simulink model "Quad_model"  (R2021b)
settings: Solver=VariableStepAuto  StartTime=0.0  StopTime=300  RelTol=1e-3
values from neighbouring files (symbols this model uses):
  A = c2d(A,1/500)    [FO_alpha.m]    (also in Model_Parameters.m = [gamma .* Wv .* (G_1+G_2) ; Wu]; wls.m = zeros(n_c,n_u))
  B = G_1+G_2    [Model_Parameters.m]    (also in wls_test.m)
  cd = 1    [Model_Parameters.m]
  G_1 = [ mot_eff,mot_eff,mot_eff,mot_eff;0,-12.8,0,12.8;2.7,0,-2.7,0;-0.115,0.115,-0.115,0.115]./conv    [Model_Parameters.m]    (also in wls_test.m)
  G_2 = [0,0,0,0;0,0,0,0;0,0,0,0;-0.06,0.06,-0.06,0.06]./conv    [Model_Parameters.m]    (also in wls_test.m)
  gamma = 10000    [Model_Parameters.m]    (also in full50.mat = [1 1 1 0]; wls_test.m = 100000000)
  gamma_o = 10000    [Model_Parameters.m]
  H_z_den = [1]    [Model_Parameters.m]
  H_z_num = [1]    [Model_Parameters.m]
  imax = 5    [Model_Parameters.m]    (also in wls_test.m)
  imax_o = 5    [Model_Parameters.m]
  M = 1    [Model_Parameters.m]
  mass = 2.339132*1    (= 2.339132)    [Model_Parameters.m]    (also in full50.mat = 3.5; pusher_effect.m)
  mot_den = [1]    [Model_Parameters.m]
  mot_num = [1]    [Model_Parameters.m]
  pseudo_g12 = pinv(G_1+G_2)    [Model_Parameters.m]    (also in wls_test.m)
  rho = 1.225    [Model_Parameters.m]    (also in full50.mat)
  Ts = 1/500    (= 0.002)    [Model_Parameters.m]
  uamax = 733    [Model_Parameters.m]    (also in wls_test.m)
  uamax_o = [0.4363,0.4363, 0]    [Model_Parameters.m]
  uamin_o = [-0.4363,-0.4363, mot_eff*4*733]    [Model_Parameters.m]
  up = [0,0,0,0]    [Model_Parameters.m]    (also in wls.m = umin; wls_test.m = [72,52,52,52])
  up_o = [0,0,0]    [Model_Parameters.m]
  v_lim = 10    [Model_Parameters.m]
  W_init = [0,0,0,0]    [Model_Parameters.m]    (also in wls_test.m)
  W_init_o = [0,0,0]    [Model_Parameters.m]
  weight = -g*mass    (= -22.94688492)    [Model_Parameters.m]
  Wu = [1, 0, 0, 0; 0, 1, 0, 0; 0, 0, 1, 0; 0, 0, 0, 1]    [Model_Parameters.m]    (also in wls_test.m = [1,1,1,1])
  Wu_o = [1,1,1]    [Model_Parameters.m]
  Wv = [100, 0, 0, 0; 0, 1000, 0, 0; 0, 0, 1000, 0; 0, 0, 0, 1 ]    [Model_Parameters.m]    (also in wls_test.m = [100,100,100,1])
  Wv_o = [1,1,1]    [Model_Parameters.m]
libraries: simulink x2, dspsrcs4 x1, sharedtransform x1, sim3dlib x1, uavsim3dlib x1, uavutilslib x1
settings Model: Creator=tomasodeponti  LastModifiedBy=Tomaso

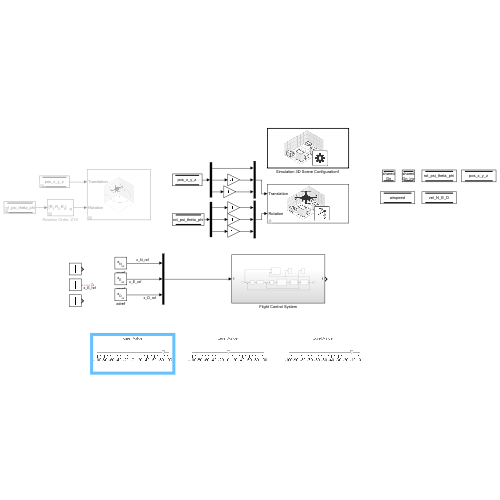
[thumbnail: Simulink's stored preview of the top-level diagram]
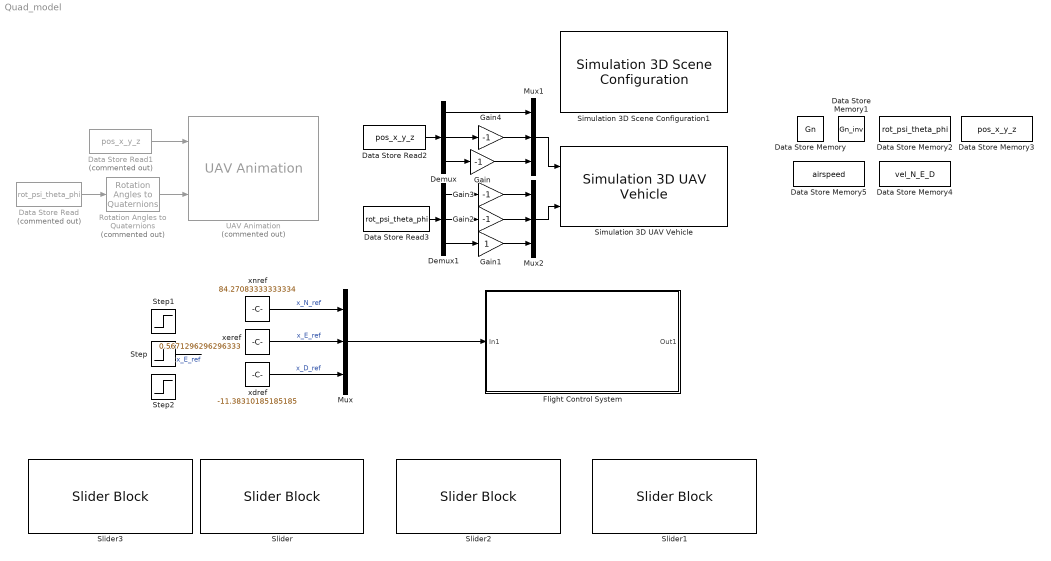
== system Quad_model ==
  Data Store Memory : DataStoreMemory  DataStoreName=Gn  ReadBeforeWriteMsg=warning  WriteAfterWriteMsg=warning  WriteAfterReadMsg=warning  InitialValue=[0,-9.81*mass,0;9.81*mass,0,0;0,0,1]  ShareAcrossModelInstances=on  ShowAdditionalParam=off  OutDataTypeStr=double  Dimensions=[3,3]
  Data Store Memory1 : DataStoreMemory  DataStoreName=Gn_inv  ReadBeforeWriteMsg=warning  WriteAfterWriteMsg=warning  WriteAfterReadMsg=warning  InitialValue=[0,-1/weight,0;1/weight,0,0;0,0,1]  ShareAcrossModelInstances=on  ShowAdditionalParam=off  OutDataTypeStr=double  Dimensions=[3,3]
  Data Store Memory2 : DataStoreMemory  DataStoreName=rot_psi_theta_phi  ReadBeforeWriteMsg=warning  WriteAfterWriteMsg=warning  WriteAfterReadMsg=warning  InitialValue=[0,0,0]  ShowAdditionalParam=off  OutDataTypeStr=double
  Data Store Memory3 : DataStoreMemory  DataStoreName=pos_x_y_z  ReadBeforeWriteMsg=warning  WriteAfterWriteMsg=warning  WriteAfterReadMsg=warning  InitialValue=[0,0,0]  ShowAdditionalParam=off  OutDataTypeStr=double
  Data Store Memory4 : DataStoreMemory  DataStoreName=vel_N_E_D  ReadBeforeWriteMsg=warning  WriteAfterWriteMsg=warning  WriteAfterReadMsg=warning  InitialValue=[0,0,0]  ShowAdditionalParam=off  OutDataTypeStr=double
  Data Store Memory5 : DataStoreMemory  DataStoreName=airspeed  ReadBeforeWriteMsg=warning  WriteAfterWriteMsg=warning  WriteAfterReadMsg=warning  InitialValue=[0]  ShowAdditionalParam=off  OutMin=[0]  OutDataTypeStr=double
  Data Store Read : DataStoreRead  Commented=on  DataStoreName=rot_psi_theta_phi  IndexOptions=Index vector (dialog)  Indices=1  OutputSizes=1
  Data Store Read1 : DataStoreRead  Commented=on  DataStoreName=pos_x_y_z  IndexOptions=Index vector (dialog)  Indices=1  OutputSizes=1
  Data Store Read2 : DataStoreRead  DataStoreName=pos_x_y_z  IndexOptions=Index vector (dialog)  Indices=1  OutputSizes=1
  Data Store Read3 : DataStoreRead  DataStoreName=rot_psi_theta_phi  IndexOptions=Index vector (dialog)  Indices=1  OutputSizes=1
  Demux : Demux  Outputs=3
  Demux1 : Demux  Outputs=3
  Flight Control System : Subsystem
  Gain{,2..4} (4 alike) : Gain  Gain=-1
  Gain1 : Gain
  Mux : Mux  Inputs=3
  Mux1 : Mux  Inputs=3
  Mux2 : Mux  Inputs=3
  Rotation Angles to Quaternions : sharedtransform/Rotation Angles to Quaternions  Commented=on  rotationOrder=ZYX  aMode=aMode
      settings: SourceProductBaseCode=AE,PW,DR,MT,UV,VE
  Simulation 3D Scene Configuration1 : sim3dlib/Simulation 3D Scene Configuration  Priority=0  ProjectFormat_internal=Default Scenes  ProjectFormat=Default Scenes  SceneDesc=US city block  ProjectName=C:\Program Files\MATLAB\R2021b\toolbox\shared\sim3d_projects\automotive_project\UE4\WindowsNoEditor\VehicleSimulation.exe  ScenePath=/Game/Maps/USCityBlock  vehTagList={'Scene Origin';'SimulinkVehicle1'}  vehTag=SimulinkVehicle1  OpVisEn=off  Ts=1/60  EnableWindow=on  EnableWeather=off  SunAltitude=40.0  SunAzimuth=90  clouds=10  wind=1  fog=0  rain=0  sensorTag=MainCamera2  sensorId=2  sensorName=MainCamera2  mountLoc=Origin  offsetFlag=off  tmountOffset=[0, 0, 0]  rmountOffset=[0, 0, 0]  HorizontalResolution=1280  VerticalResolution=720  HorizontalFOV=60  mountPoint=[0 0 0]  mountOrientation=[0 0 0]  aMode=4  ID=2
      settings: SourceProductBaseCode=AE,DR,UV,VE
  Simulation 3D UAV Vehicle : uavsim3dlib/Simulation 3D UAV Vehicle  Priority=-1  Mesh=Quadrotor  MeshPath=/MathWorksUAVContent/UAVs/HexaRotorUAV/HexaRotor.HexaRotor  Color=Black  ActorName=SimulinkVehicle1  InitialTranslation=[0 0 5]  InitialRotation=[0 0 0]  SampleTime=-1  ActorType=SimulinkVehicle  ID=1  aMode=4  ActorTag=SimulinkVehicle1
      settings: SourceProductBaseCode=UV
  Slider : SliderBlock  ScaleMin=-100
  Slider1 : SliderBlock  ScaleMin=-100  ScaleMax=0
  Slider2 : SliderBlock  ScaleMin=-100
  Slider3 : SliderBlock  ScaleMin=-3.14  ScaleMax=3.14
  Step : Step  Time=3  After=50  SampleTime=0
  Step1 : Step  Time=3  After=100  SampleTime=0
  Step2 : Step  Time=4  After=-25  SampleTime=0
  UAV Animation : uavutilslib/UAV Animation  Commented=on  UAVType=Multirotor  UAVSize=1  InertialZDirection=Down  SampleTime=-1
      settings: SourceProductBaseCode=UV
  xdref : Constant  Value=-11.38310185185185  SampleTime=Ts
      mask Display: disp('x_{D_{ref}}','texmode','on')
  xeref : Constant  Value=0.5671296296296333  SampleTime=Ts
      mask Display: disp('x_{E_{ref}}','texmode','on')
  xnref : Constant  Value=84.27083333333334  SampleTime=Ts
      mask Display: disp('x_{N_{ref}}','texmode','on')
  wires:
  Data Store Read1/1 -> UAV Animation/1
  Data Store Read/1 -> Rotation Angles to Quaternions/1
  Rotation Angles to Quaternions/1 -> UAV Animation/2
  xdref/1 -> Mux/3  "x_D_ref"
  xnref/1 -> Mux/1  "x_N_ref"
  Mux/1 -> Flight Control System/1(In1)
  xeref/1 -> Mux/2  "x_E_ref"
  Step/1 -> ?  "x_E_ref"
  Data Store Read2/1 -> Demux/1
  Mux1/1 -> Simulation 3D UAV Vehicle/1
  Demux/3 -> Gain/1
  Gain/1 -> Mux1/3
  Data Store Read3/1 -> Demux1/1
  Demux1/3 -> Gain1/1
  Gain1/1 -> Mux2/3
  Mux2/1 -> Simulation 3D UAV Vehicle/2
  Demux1/2 -> Gain2/1
  Gain2/1 -> Mux2/2
  Demux1/1 -> Gain3/1
  Gain3/1 -> Mux2/1
  Demux/2 -> Gain4/1
  Gain4/1 -> Mux1/2
  Demux/1 -> Mux1/1

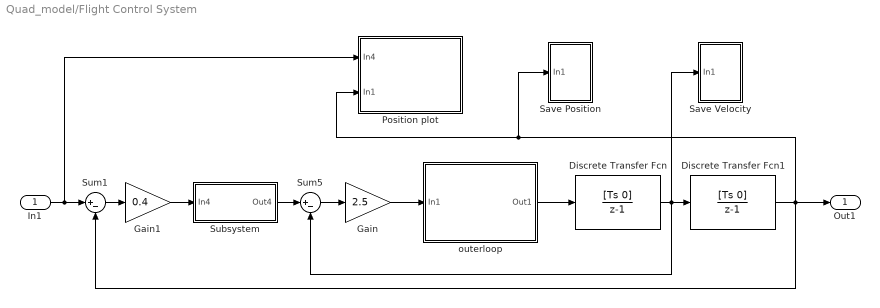
== system Quad_model/Flight Control System ==
  In1 : Inport
  Discrete Transfer Fcn : DiscreteTransferFcn  Numerator=[Ts 0]  Denominator=[1 -1]
  Discrete Transfer Fcn1 : DiscreteTransferFcn  Numerator=[Ts 0]  Denominator=[1 -1]
  Gain : Gain  Gain=2.5
      mask Display: disp('K_{u}','texmode','on')
  Gain1 : Gain  Gain=0.4
      mask Display: disp('K_\xi','texmode','on')
  Position plot : Subsystem
  Save Position : Subsystem
  Save Velocity : Subsystem
  Subsystem : Subsystem
      mask Display: disp('Velocity lim')
  Sum1 : Sum  Inputs=|+-
  Sum5 : Sum  Inputs=|+-
  outerloop : Subsystem
  Out1 : Outport
  wires:
  outerloop/1(Out1) -> Discrete Transfer Fcn/1
  Discrete Transfer Fcn1/1 -> Position plot/2(In1), Save Position/1(In1), Out1/1, Sum1/2
  Sum5/1 -> Gain/1
  Gain/1 -> outerloop/1(In1)
  Discrete Transfer Fcn/1 -> Save Velocity/1(In1), Sum5/2, Discrete Transfer Fcn1/1
  In1/1 -> Position plot/1(In4), Sum1/1
  Gain1/1 -> Subsystem/1(In4)
  Subsystem/1(Out4) -> Sum5/1
  Sum1/1 -> Gain1/1

== system Quad_model/Flight Control System/Position plot ==
  In4 : Inport
  In1 : Inport  Port=2
  Demux : Demux  Outputs=3
  Demux1 : Demux  Outputs=3
  Mux : Mux  Inputs=2
  Mux1 : Mux  Inputs=2
  Mux3 : Mux  Inputs=2
  Position Plotter : Scope  NumInputPorts=3
  wires:
  Demux/3 -> Mux3/1  "x_D"
  Demux/2 -> Mux1/1  "x_E"
  In1/1 -> Demux/1
  Mux/1 -> Position Plotter/1
  Demux/1 -> Mux/1  "x_N"
  Mux1/1 -> Position Plotter/2
  Mux3/1 -> Position Plotter/3
  In4/1 -> Demux1/1
  Demux1/1 -> Mux/2  "x_N_ref"
  Demux1/2 -> Mux1/2  "x_E_ref"
  Demux1/3 -> Mux3/2  "x_D_ref"

== system Quad_model/Flight Control System/Save Position ==
  In1 : Inport
  Data Store Write : DataStoreWrite  DataStoreName=pos_x_y_z  IndexOptions=Index vector (dialog)  Indices=1  OutputSizes=1
  Demux : Demux  Outputs=3
  Mux4 : Mux  Inputs=3
  wires:
  Mux4/1 -> Data Store Write/1
  Demux/2 -> Mux4/2
  Demux/1 -> Mux4/1
  Demux/3 -> Mux4/3
  In1/1 -> Demux/1

== system Quad_model/Flight Control System/Save Velocity ==
  In1 : Inport
  Data Store Write : DataStoreWrite  DataStoreName=vel_N_E_D  IndexOptions=Index vector (dialog)  Indices=1  OutputSizes=1
  Data Store Write1 : DataStoreWrite  DataStoreName=airspeed  IndexOptions=Index vector (dialog)  Indices=1  OutputSizes=1
  Demux : Demux  Outputs=3
  Dot Product : DotProduct  InputSameDT=on  OutDataTypeStr=Inherit: Inherit via internal rule
  Mux : Mux  Inputs=2
  Mux4 : Mux  Inputs=3
  Scope : Scope
  Square Root : Sqrt  SaturateOnIntegerOverflow=on
  wires:
  Mux4/1 -> Data Store Write/1
  Demux/2 -> Mux/2, Mux4/2
  Demux/1 -> Mux/1, Mux4/1
  Demux/3 -> Mux4/3
  In1/1 -> Demux/1
  Dot Product/1 -> Square Root/1
  Square Root/1 -> Scope/1, Data Store Write1/1
  Mux/1 -> Dot Product/2, Dot Product/1

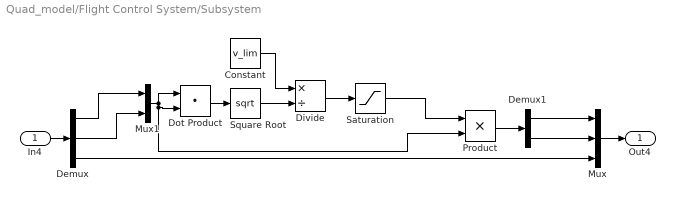
== system Quad_model/Flight Control System/Subsystem ==
  In4 : Inport
  Constant : Constant  Value=v_lim
  Demux : Demux  Outputs=3
  Demux1 : Demux  Outputs=2
  Divide : Product  Inputs=*/
  Dot Product : DotProduct  InputSameDT=on  OutDataTypeStr=Inherit: Inherit via internal rule
  Mux : Mux  Inputs=3
  Mux1 : Mux  Inputs=2
  Product : Product
  Saturation : Saturate  UpperLimit=1  LowerLimit=0
  Square Root : Sqrt  SaturateOnIntegerOverflow=on
  Out4 : Outport
  wires:
  In4/1 -> Demux/1
  Mux/1 -> Out4/1
  Constant/1 -> Divide/1
  Demux/3 -> Mux/3
  Demux/1 -> Mux1/1
  Demux/2 -> Mux1/2
  Dot Product/1 -> Square Root/1
  Mux1/1 -> Product/2, Dot Product/2, Dot Product/1
  Square Root/1 -> Divide/2
  Divide/1 -> Saturation/1
  Product/1 -> Demux1/1
  Demux1/1 -> Mux/1
  Demux1/2 -> Mux/2
  Saturation/1 -> Product/1

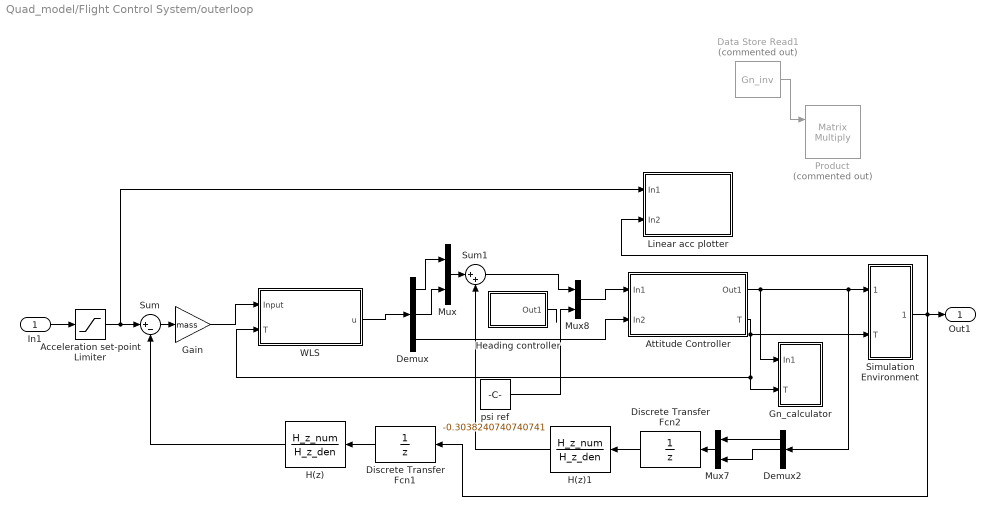
== system Quad_model/Flight Control System/outerloop ==
  In1 : Inport
  Acceleration set-point Limiter : Saturate  UpperLimit=[3,3,3]  LowerLimit=[-3,-3,-3]
  Attitude Controller : Subsystem
  Data Store Read1 : DataStoreRead  Commented=on  DataStoreName=Gn_inv  SampleTime=Ts  IndexOptions=Index vector (dialog)  Indices=1  OutputSizes=1
  Demux : Demux  Outputs=3
  Demux2 : Demux  Outputs=3
  Discrete Transfer Fcn1 : DiscreteTransferFcn  Denominator=[1 0]
  Discrete Transfer Fcn2 : DiscreteTransferFcn  Denominator=[1 0]
  Gain : Gain  Gain=mass
  Gn_calculator : Subsystem
  H(z) : DiscreteTransferFcn  Numerator=H_z_num  Denominator=H_z_den  DenCoefDataTypeStr=int16
      mask Display: disp('H(z)')
  H(z)1 : DiscreteTransferFcn  Numerator=H_z_num  Denominator=H_z_den  DenCoefDataTypeStr=int16
      mask Display: disp('H(z)')
  Heading controller : Subsystem
  Linear acc plotter : Subsystem
  Mux : Mux  Inputs=2
  Mux7 : Mux  Inputs=2
  Mux8 : Mux  Inputs=2
  Product : Product  Commented=on  Multiplication=Matrix(*)
      mask Display: disp('G(\eta_0,T_0)^+','texmode','on')
  Simulation Environment : Subsystem
  Sum : Sum  Inputs=|+-
  Sum1 : Sum  Inputs=|++
  WLS : Subsystem
  psi ref : Constant  Value=-0.3038240740740741
  Out1 : Outport
  wires:
  Mux7/1 -> Discrete Transfer Fcn2/1
  Data Store Read1/1 -> Product/1
  WLS/1(u) -> Demux/1
  Discrete Transfer Fcn2/1 -> H(z)1/1
  Mux/1 -> Sum1/1
  Demux/3 -> Attitude Controller/2(In2)
  Attitude Controller/1(Out1) -> Gn_calculator/1(In1), Demux2/1, Simulation Environment/1(In1)
  H(z)/1 -> Sum/2
  Discrete Transfer Fcn1/1 -> H(z)/1
  Gain/1 -> WLS/1(Input)
  Demux/2 -> Mux/2
  Sum/1 -> Gain/1
  Attitude Controller/2(T) -> WLS/2(T), Gn_calculator/2(T), Simulation Environment/2(T)
  Sum1/1 -> Mux8/1
  Mux8/1 -> Attitude Controller/1(In1)
  Demux2/1 -> Mux7/1
  H(z)1/1 -> Sum1/2
  Demux/1 -> Mux/1
  Simulation Environment/1(Out1) -> Discrete Transfer Fcn1/1, Out1/1, Linear acc plotter/2(In2)
  Demux2/2 -> Mux7/2
  Acceleration set-point Limiter/1 -> Linear acc plotter/1(In1), Sum/1
  In1/1 -> Acceleration set-point Limiter/1
  psi ref/1 -> Mux8/2
  Heading controller/1(Out1) -> ?

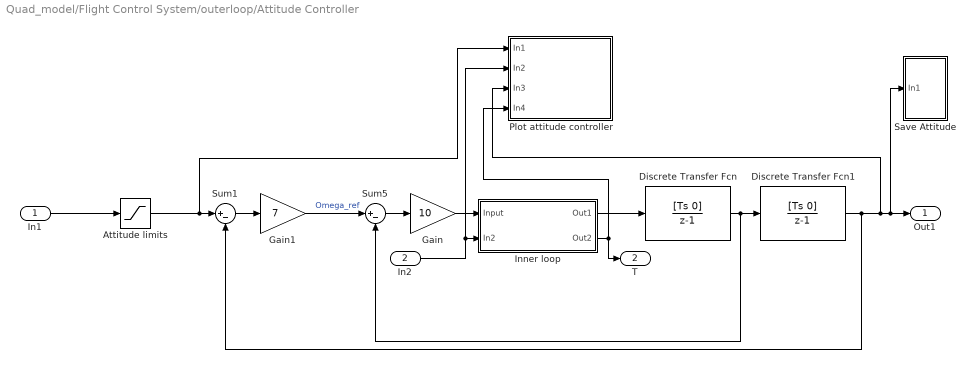
== system Quad_model/Flight Control System/outerloop/Attitude Controller ==
  In1 : Inport
  In2 : Inport  Port=2
  Attitude limits : Saturate  UpperLimit=[25,25,180]*pi/180  LowerLimit=[-25,-25,-180]*pi/180
  Discrete Transfer Fcn : DiscreteTransferFcn  Numerator=[Ts 0]  Denominator=[1 -1]
  Discrete Transfer Fcn1 : DiscreteTransferFcn  Numerator=[Ts 0]  Denominator=[1 -1]
  Gain : Gain  Gain=10
      mask Display: disp('K_\Omega','texmode','on')
  Gain1 : Gain  Gain=7
      mask Display: disp('K_\eta','texmode','on')
  Inner loop : Subsystem
  Plot attitude controller : Subsystem
  Save Attitude : Subsystem
  Sum1 : Sum  Inputs=|+-
  Sum5 : Sum  Inputs=|+-
  Out1 : Outport
  T : Outport  Port=2
  wires:
  Gain1/1 -> Sum5/1  "Omega_ref"
  Sum5/1 -> Gain/1
  Sum1/1 -> Gain1/1
  Discrete Transfer Fcn/1 -> Sum5/2, Discrete Transfer Fcn1/1
  Gain/1 -> Inner loop/1(Input)
  Inner loop/1(Out1) -> Discrete Transfer Fcn/1
  Discrete Transfer Fcn1/1 -> Plot attitude controller/3(In3), Save Attitude/1(In1), Out1/1, Sum1/2
  Inner loop/2(Out2) -> T/1, Plot attitude controller/4(In4)
  In2/1 -> Plot attitude controller/2(In2), Inner loop/2(In2)
  Attitude limits/1 -> Plot attitude controller/1(In1), Sum1/1
  In1/1 -> Attitude limits/1

== system Quad_model/Flight Control System/outerloop/Gn_calculator ==
  In1 : Inport
  T : Inport  Port=2
  Constant : Constant  Value=weight
  Demux : Demux  Outputs=3
  Gn : MATLAB Function  TreatAsAtomicUnit=on
  Gn_inv : MATLAB Function  TreatAsAtomicUnit=on
  wires:
  Demux/1 -> Gn_inv/2(phi), Gn/2(phi)
  In1/1 -> Demux/1
  T/1 -> Gn_inv/1(T), Gn/1(T)
  Demux/2 -> Gn_inv/3(theta), Gn/3(theta)
  Demux/3 -> Gn_inv/4(psi), Gn/4(psi)

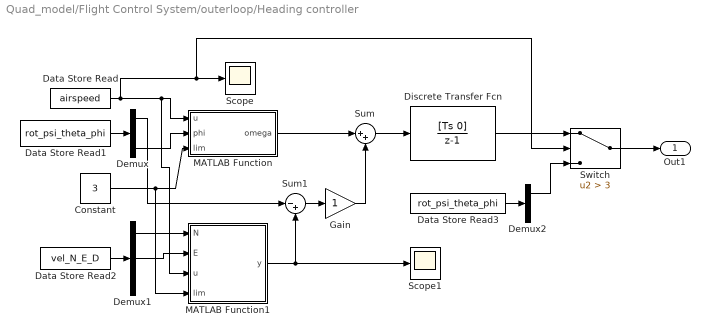
== system Quad_model/Flight Control System/outerloop/Heading controller ==
  Constant : Constant  Value=3
  Data Store Read : DataStoreRead  DataStoreName=airspeed  IndexOptions=Index vector (dialog)  Indices=1  OutputSizes=1
  Data Store Read1 : DataStoreRead  DataStoreName=rot_psi_theta_phi  IndexOptions=Index vector (dialog)  Indices=1  OutputSizes=1
  Data Store Read2 : DataStoreRead  DataStoreName=vel_N_E_D  IndexOptions=Index vector (dialog)  Indices=1  OutputSizes=1
  Data Store Read3 : DataStoreRead  DataStoreName=rot_psi_theta_phi  IndexOptions=Index vector (dialog)  Indices=1  OutputSizes=1
  Demux : Demux  Outputs=3
  Demux1 : Demux  Outputs=3
  Demux2 : Demux  Outputs=3
  Discrete Transfer Fcn : DiscreteTransferFcn  Numerator=[Ts 0]  Denominator=[1 -1]
  Gain : Gain
  MATLAB Function : MATLAB Function  TreatAsAtomicUnit=on
  MATLAB Function1 : MATLAB Function  TreatAsAtomicUnit=on
  Scope : Scope
  Scope1 : Scope
  Sum : Sum  Inputs=|++
  Sum1 : Sum  Inputs=|-+
  Switch : Switch  Criteria=u2 > Threshold  Threshold=3
  Out1 : Outport
  wires:
  Data Store Read1/1 -> Demux/1
  Demux/3 -> MATLAB Function/2(phi)
  Data Store Read/1 -> Switch/2, Scope/1, MATLAB Function1/3(u), MATLAB Function/1(u)
  Data Store Read2/1 -> Demux1/1
  Demux1/1 -> MATLAB Function1/1(N)
  Demux1/2 -> MATLAB Function1/2(E)
  Switch/1 -> Out1/1
  Sum/1 -> Discrete Transfer Fcn/1
  MATLAB Function/1(omega) -> Sum/1
  Gain/1 -> Sum/2
  MATLAB Function1/1(y) -> Sum1/2, Scope1/1
  Demux/1 -> Sum1/1
  Sum1/1 -> Gain/1
  Constant/1 -> MATLAB Function/3(lim), MATLAB Function1/4(lim)
  Discrete Transfer Fcn/1 -> Switch/1
  Data Store Read3/1 -> Demux2/1
  Demux2/1 -> Switch/3

== system Quad_model/Flight Control System/outerloop/Linear acc plotter ==
  In1 : Inport
  In2 : Inport  Port=2
  Constant1 : Constant  Value=0  SampleTime=Ts
      mask Display: disp('a_{N_{ref}}','texmode','on')
  Constant2 : Constant  Value=0  SampleTime=Ts
      mask Display: disp('a_{E_{ref}}','texmode','on')
  Constant3 : Constant  Value=0  SampleTime=Ts
      mask Display: disp('a_{D_{ref}}','texmode','on')
  Demux1 : Demux  Outputs=3
  Demux2 : Demux  Outputs=3
  Mux1 : Mux  Inputs=2
  Mux2 : Mux  Inputs=3
  Mux3 : Mux  Inputs=2
  Mux4 : Mux  Inputs=2
  Scope : Scope  NumInputPorts=3
  wires:
  Demux1/3 -> Mux4/1  "a_D"
  Mux1/1 -> Scope/1
  In2/1 -> Demux1/1
  Mux3/1 -> Scope/2
  Mux4/1 -> Scope/3
  Demux1/2 -> Mux3/1  "a_E"
  Demux1/1 -> Mux1/1  "a_N"
  Constant2/1 -> Mux2/2  "a_E_ref"
  Constant1/1 -> Mux2/1  "a_N_ref"
  Constant3/1 -> Mux2/3  "a_D_ref"
  In1/1 -> Demux2/1
  Demux2/1 -> Mux1/2  "a_N_ref"
  Demux2/2 -> Mux3/2  "a_E_ref"
  Demux2/3 -> Mux4/2  "a_D_ref"

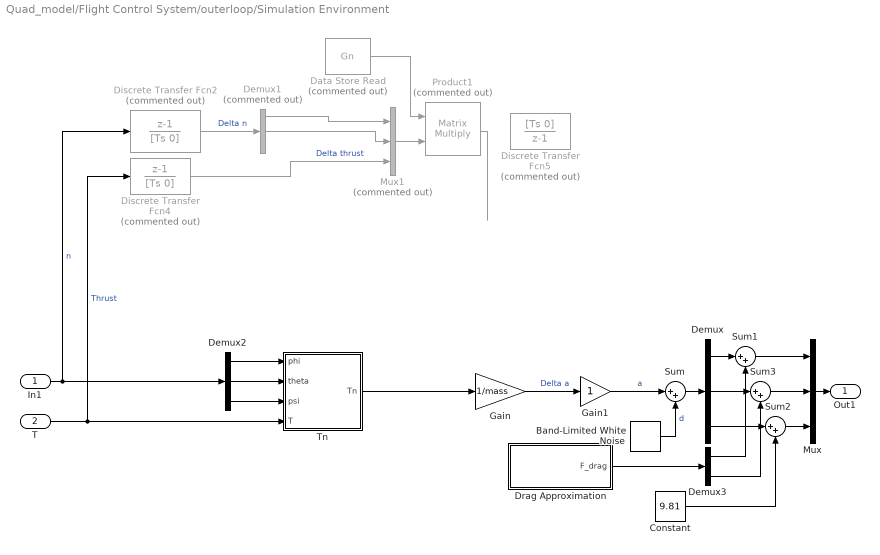
== system Quad_model/Flight Control System/outerloop/Simulation Environment ==
  In1 : Inport
  T : Inport  Port=2
  Band-Limited White Noise : simulink/Sources/Band-Limited White Noise  Cov=[0.00000001]  Ts=Ts  seed=[23341]
  Constant : Constant  Value=9.81
  Data Store Read : DataStoreRead  Commented=on  DataStoreName=Gn  IndexOptions=Index vector (dialog)  Indices=1  OutputSizes=1
  Demux : Demux  Outputs=3
  Demux1 : Demux  Commented=on  Outputs=3
  Demux2 : Demux  Outputs=3
  Demux3 : Demux  Outputs=2
  Discrete Transfer Fcn2 : DiscreteTransferFcn  Commented=on  Numerator=[1 -1]  Denominator=[Ts 0]
  Discrete Transfer Fcn4 : DiscreteTransferFcn  Commented=on  Numerator=[1 -1]  Denominator=[Ts 0]
  Discrete Transfer Fcn5 : DiscreteTransferFcn  Commented=on  Numerator=[Ts 0]  Denominator=[1 -1]
  Drag Approximation : Subsystem
  Gain : Gain  Gain=1/mass
  Gain1 : Gain
  Mux : Mux  Inputs=3
  Mux1 : Mux  Commented=on  Inputs=3
  Product1 : Product  Commented=on  Multiplication=Matrix(*)
      mask Display: disp('G(\eta_0,T_0)','texmode','on')
  Sum{,1..3} (4 alike) : Sum  Inputs=|++
  Tn : MATLAB Function  TreatAsAtomicUnit=on
  Out1 : Outport
  wires:
  In1/1 -> Discrete Transfer Fcn2/1, Demux2/1  "n"
  Data Store Read/1 -> Product1/1
  Mux1/1 -> Product1/2
  Demux1/1 -> Mux1/1
  Demux1/2 -> Mux1/2
  Discrete Transfer Fcn2/1 -> Demux1/1  "Delta n"
  Gain/1 -> Gain1/1  "Delta a"
  Gain1/1 -> Sum/1  "a"
  Product1/1 -> ?
  T/1 -> Discrete Transfer Fcn4/1, Tn/4(T)  "Thrust"
  Discrete Transfer Fcn4/1 -> Mux1/3  "Delta thrust"
  Band-Limited White Noise/1 -> Sum/2  "d"
  Demux2/1 -> Tn/1(phi)
  Demux2/2 -> Tn/2(theta)
  Demux2/3 -> Tn/3(psi)
  Tn/1(Tn) -> Gain/1
  Drag Approximation/1(F_drag) -> Demux3/1
  Sum/1 -> Demux/1
  Sum3/1 -> Mux/2
  Mux/1 -> Out1/1
  Demux/3 -> Sum2/1
  Sum2/1 -> Mux/3
  Sum1/1 -> Mux/1
  Demux/1 -> Sum1/1
  Demux/2 -> Sum3/1
  Demux3/1 -> Sum1/2
  Demux3/2 -> Sum3/2
  Constant/1 -> Sum2/2

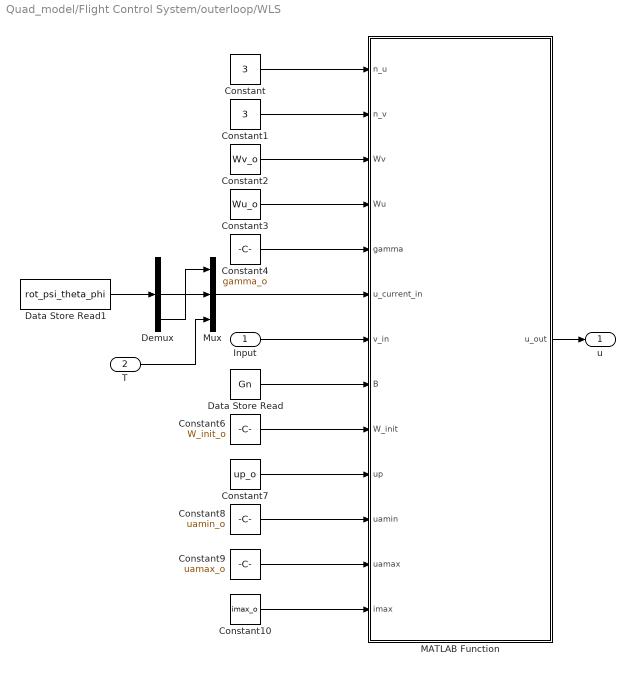
== system Quad_model/Flight Control System/outerloop/WLS ==
  Input : Inport
  T : Inport  Port=2
  Constant : Constant  Value=3
  Constant1 : Constant  Value=3
  Constant10 : Constant  Value=imax_o
  Constant2 : Constant  Value=Wv_o
  Constant3 : Constant  Value=Wu_o
  Constant4 : Constant  Value=gamma_o
  Constant6 : Constant  Value=W_init_o
  Constant7 : Constant  Value=up_o
  Constant8 : Constant  Value=uamin_o
  Constant9 : Constant  Value=uamax_o
  Data Store Read : DataStoreRead  DataStoreName=Gn  IndexOptions=Index vector (dialog)  Indices=1  OutputSizes=1
  Data Store Read1 : DataStoreRead  DataStoreName=rot_psi_theta_phi  IndexOptions=Index vector (dialog)  Indices=1  OutputSizes=1
  Demux : Demux  Outputs=3
  MATLAB Function : MATLAB Function  TreatAsAtomicUnit=on
  Mux : Mux  Inputs=3
  u : Outport
  wires:
  Constant8/1 -> MATLAB Function/11(uamin)
  Constant4/1 -> MATLAB Function/5(gamma)
  Constant/1 -> MATLAB Function/1(n_u)
  MATLAB Function/1(u_out) -> u/1
  Data Store Read/1 -> MATLAB Function/8(B)
  Constant9/1 -> MATLAB Function/12(uamax)
  Constant6/1 -> MATLAB Function/9(W_init)
  Constant10/1 -> MATLAB Function/13(imax)
  Constant1/1 -> MATLAB Function/2(n_v)
  Constant2/1 -> MATLAB Function/3(Wv)
  Constant3/1 -> MATLAB Function/4(Wu)
  Constant7/1 -> MATLAB Function/10(up)
  Mux/1 -> MATLAB Function/6(u_current_in)
  Input/1 -> MATLAB Function/7(v_in)
  Data Store Read1/1 -> Demux/1
  Demux/3 -> Mux/1
  Demux/2 -> Mux/2
  T/1 -> Mux/3

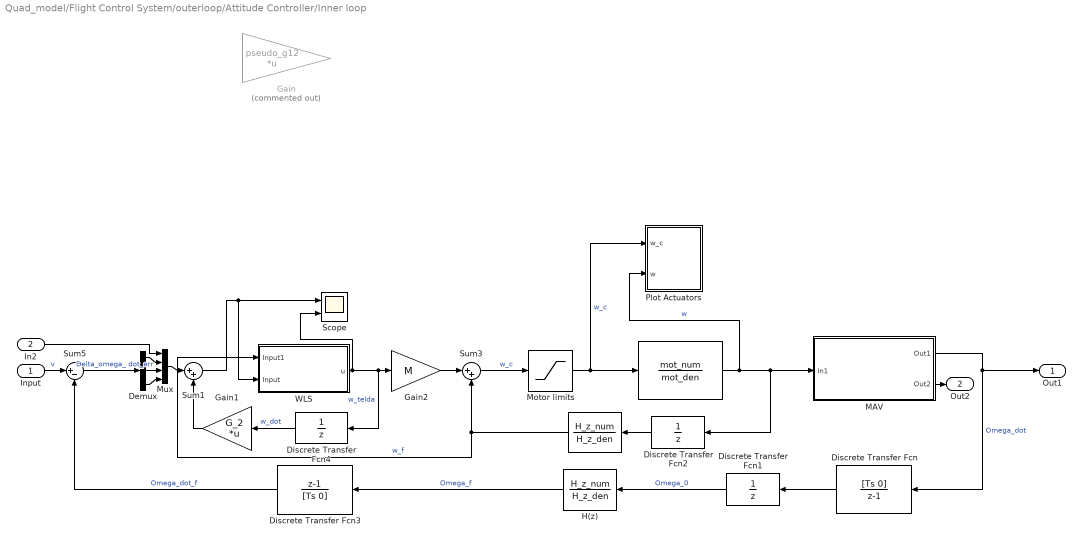
== system Quad_model/Flight Control System/outerloop/Attitude Controller/Inner loop ==
  Input : Inport  PortDimensions=3
  In2 : Inport  Port=2
  " " : DiscreteTransferFcn  Numerator=H_z_num  Denominator=H_z_den  DenCoefDataTypeStr=int16
      mask Display: disp('H(z)')
  "  " : DiscreteTransferFcn  Numerator=mot_num  Denominator=mot_den  DenCoefDataTypeStr=int16
      mask Display: disp('A(z)')
  Demux : Demux  Outputs=3
  Discrete Transfer Fcn : DiscreteTransferFcn  Numerator=[Ts 0]  Denominator=[1 -1]
  Discrete Transfer Fcn1 : DiscreteTransferFcn  Denominator=[1 0]
  Discrete Transfer Fcn2 : DiscreteTransferFcn  Denominator=[1 0]
  Discrete Transfer Fcn3 : DiscreteTransferFcn  Numerator=[1 -1]  Denominator=[Ts 0]
  Discrete Transfer Fcn4 : DiscreteTransferFcn  Denominator=[1 0]
  Gain : Gain  Commented=on  Gain=pseudo_g12  Multiplication=Matrix(K*u)
      mask Display: disp('(G1+G2)^+','texmode','on')
  Gain1 : Gain  Gain=G_2  Multiplication=Matrix(K*u)
      mask Display: disp('G2')
  Gain2 : Gain  Gain=M
      mask Display: disp('M')
  H(z) : DiscreteTransferFcn  Numerator=H_z_num  Denominator=H_z_den  DenCoefDataTypeStr=int16
      mask Display: disp('H(z)')
  MAV : Subsystem
      mask Display:
      | %image('C:\Users\Tomaso\Pictures\Screenshots\Screenshot 2021-12-02 165056.png'); % Use "Edit Image" on toolstrip to change.
      | disp('MAV')
  Motor limits : Saturate  UpperLimit=733  LowerLimit=52
  Mux : Mux
  Plot Actuators : Subsystem
  Scope : Scope  NumInputPorts=2
  Sum1 : Sum  Inputs=|++
  Sum3 : Sum  Inputs=|++
  Sum5 : Sum  Inputs=|+-
  WLS : Subsystem
  Out1 : Outport  PortDimensions=3
  Out2 : Outport  Port=2
  wires:
  "  "/1 -> Plot Actuators/2(w), Discrete Transfer Fcn2/1, MAV/1(In1)  "w"
  Discrete Transfer Fcn/1 -> Discrete Transfer Fcn1/1
  Discrete Transfer Fcn1/1 -> H(z)/1  "Omega_0"
  Discrete Transfer Fcn2/1 -> " "/1
  Motor limits/1 -> Plot Actuators/1(w_c), "  "/1  "w_c"
  " "/1 -> Sum3/2, WLS/1(Input1)  "w_f"
  H(z)/1 -> Discrete Transfer Fcn3/1  "Omega_f"
  Discrete Transfer Fcn3/1 -> Sum5/2  "Omega_dot_f"
  WLS/1(u) -> Scope/2, Discrete Transfer Fcn4/1, Gain2/1  "w_telda"
  Sum5/1 -> Demux/1  "Delta_omega_ dot_err"
  Sum1/1 -> Scope/1, WLS/2(Input)
  Discrete Transfer Fcn4/1 -> Gain1/1  "w_dot"
  Gain1/1 -> Sum1/2
  Input/1 -> Sum5/1  "v"
  Gain2/1 -> Sum3/1
  Sum3/1 -> Motor limits/1  "w_c"
  MAV/1(Out1) -> Discrete Transfer Fcn/1, Out1/1  "Omega_dot"
  In2/1 -> Mux/1
  Mux/1 -> Sum1/1
  Demux/1 -> Mux/2
  Demux/2 -> Mux/3
  Demux/3 -> Mux/4
  MAV/2(Out2) -> Out2/1

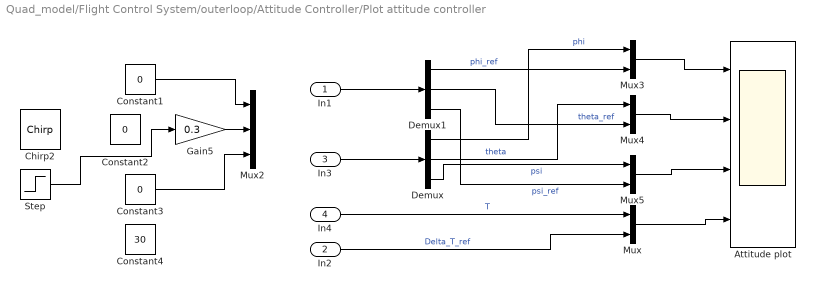
== system Quad_model/Flight Control System/outerloop/Attitude Controller/Plot attitude controller ==
  In1 : Inport
  In2 : Inport  Port=2
  In3 : Inport  Port=3
  In4 : Inport  Port=4
  Attitude plot : Scope  NumInputPorts=4
  Chirp2 : dspsrcs4/Chirp  sweep=Linear  mode=Unidirectional  f0=0.1  f1=0.5  t1=1  Tsweep=10  phase=0  Ts=Ts  spf=1  datatype=Double  OutputFrames=off
  Constant1 : Constant  Value=0
      mask Display: disp('\phi_{ref}','texmode','on')
  Constant2 : Constant  Value=0
      mask Display: disp('\theta_{ref}','texmode','on')
  Constant3 : Constant  Value=0
      mask Display: disp('\psi_{ref}','texmode','on')
  Constant4 : Constant  Value=30
      mask Display: disp('\Delta T','texmode','on')
  Demux : Demux  Outputs=3
  Demux1 : Demux  Outputs=3
  Gain5 : Gain  Gain=0.3
  Mux{,3..5} (4 alike) : Mux  Inputs=2
  Mux2 : Mux  Inputs=3
  Step : Step  SampleTime=0
  wires:
  In4/1 -> Mux/1  "T"
  In3/1 -> Demux/1
  Mux4/1 -> Attitude plot/2
  Demux1/1 -> Mux3/2  "phi_ref"
  Demux/2 -> Mux4/1  "theta"
  In1/1 -> Demux1/1
  Demux/3 -> Mux5/1  "psi"
  Demux1/3 -> Mux5/2  "psi_ref"
  Demux1/2 -> Mux4/2  "theta_ref"
  Demux/1 -> Mux3/1  "phi"
  Mux3/1 -> Attitude plot/1
  Mux5/1 -> Attitude plot/3
  Constant1/1 -> Mux2/1
  Step/1 -> Gain5/1
  Constant3/1 -> Mux2/3
  Gain5/1 -> Mux2/2
  Mux/1 -> Attitude plot/4
  In2/1 -> Mux/2  "Delta_T_ref"

== system Quad_model/Flight Control System/outerloop/Attitude Controller/Save Attitude ==
  In1 : Inport
  Data Store Write : DataStoreWrite  DataStoreName=rot_psi_theta_phi  IndexOptions=Index vector (dialog)  Indices=1  OutputSizes=1
  Demux : Demux  Outputs=3
  Mux : Mux  Inputs=3
  wires:
  In1/1 -> Demux/1
  Mux/1 -> Data Store Write/1
  Demux/3 -> Mux/1
  Demux/1 -> Mux/3
  Demux/2 -> Mux/2

== system Quad_model/Flight Control System/outerloop/Simulation Environment/Drag Approximation ==
  Constant : Constant  Value=cd
  Constant1 : Constant  Value=rho
  Constant2 : Constant  Value=A
  Data Store Read : DataStoreRead  DataStoreName=airspeed  IndexOptions=Index vector (dialog)  Indices=1  OutputSizes=1
  Data Store Read2 : DataStoreRead  DataStoreName=vel_N_E_D  IndexOptions=Index vector (dialog)  Indices=1  OutputSizes=1
  Demux1 : Demux  Outputs=3
  MATLAB Function : MATLAB Function  TreatAsAtomicUnit=on
  MATLAB Function1 : MATLAB Function  TreatAsAtomicUnit=on
  F_drag : Outport
  wires:
  Data Store Read2/1 -> Demux1/1
  Demux1/1 -> MATLAB Function1/1(N)
  Demux1/2 -> MATLAB Function1/2(E)
  Data Store Read/1 -> MATLAB Function/3(u)
  MATLAB Function1/1(y) -> MATLAB Function/5(trj)
  MATLAB Function/1(F_drag) -> F_drag/1
  Constant/1 -> MATLAB Function/1(cd)
  Constant1/1 -> MATLAB Function/2(rho)
  Constant2/1 -> MATLAB Function/4(A)

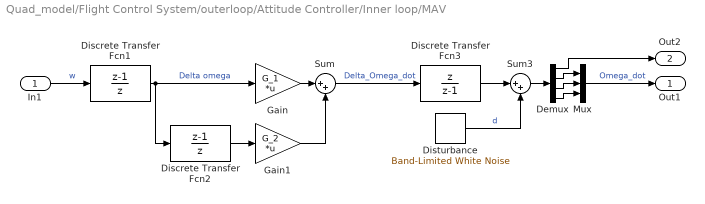
== system Quad_model/Flight Control System/outerloop/Attitude Controller/Inner loop/MAV ==
  In1 : Inport  PortDimensions=4
  Demux : Demux
  Discrete Transfer Fcn1 : DiscreteTransferFcn  Numerator=[1 -1]  Denominator=[1 0]
  Discrete Transfer Fcn2 : DiscreteTransferFcn  Numerator=[1 -1]  Denominator=[1 0]
  Discrete Transfer Fcn3 : DiscreteTransferFcn  Numerator=[1 0]  Denominator=[1 -1]
  Disturbance : simulink/Sources/Band-Limited White Noise  Cov=[0.00000001]  Ts=Ts  seed=[23341]
  Gain : Gain  Gain=G_1  Multiplication=Matrix(K*u)
      mask Display: disp('G1')
  Gain1 : Gain  Gain=G_2  Multiplication=Matrix(K*u)
      mask Display: disp('G2')
  Mux : Mux  Inputs=3
  Sum : Sum  Inputs=|++
  Sum3 : Sum  Inputs=|++
  Out1 : Outport  PortDimensions=3
  Out2 : Outport  Port=2
  wires:
  In1/1 -> Discrete Transfer Fcn1/1  "w"
  Discrete Transfer Fcn1/1 -> Discrete Transfer Fcn2/1, Gain/1  "Delta omega"
  Discrete Transfer Fcn2/1 -> Gain1/1
  Gain/1 -> Sum/1
  Gain1/1 -> Sum/2
  Sum/1 -> Discrete Transfer Fcn3/1  "Delta_Omega_dot"
  Discrete Transfer Fcn3/1 -> Sum3/1
  Disturbance/1 -> Sum3/2  "d"
  Mux/1 -> Out1/1  "Omega_dot"
  Sum3/1 -> Demux/1
  Demux/4 -> Mux/3
  Demux/3 -> Mux/2
  Demux/2 -> Mux/1
  Demux/1 -> Out2/1

== system Quad_model/Flight Control System/outerloop/Attitude Controller/Inner loop/Plot Actuators ==
  w_c : Inport
  w : Inport  Port=2
  Demux : Demux
  Demux1 : Demux
  Motor State : Scope  NumInputPorts=4
  Mux{,1..3} (4 alike) : Mux  Inputs=2
  wires:
  Demux1/3 -> Mux1/2
  w_c/1 -> Demux/1
  Demux1/4 -> Mux3/2
  Demux/2 -> Mux2/1
  w/1 -> Demux1/1
  Demux/4 -> Mux3/1
  Mux/1 -> Motor State/1  "mot1"
  Demux/3 -> Mux1/1
  Demux1/1 -> Mux/2
  Demux/1 -> Mux/1
  Mux1/1 -> Motor State/3  "mot3"
  Demux1/2 -> Mux2/2
  Mux2/1 -> Motor State/2  "mot2"
  Mux3/1 -> Motor State/4  "mot4"

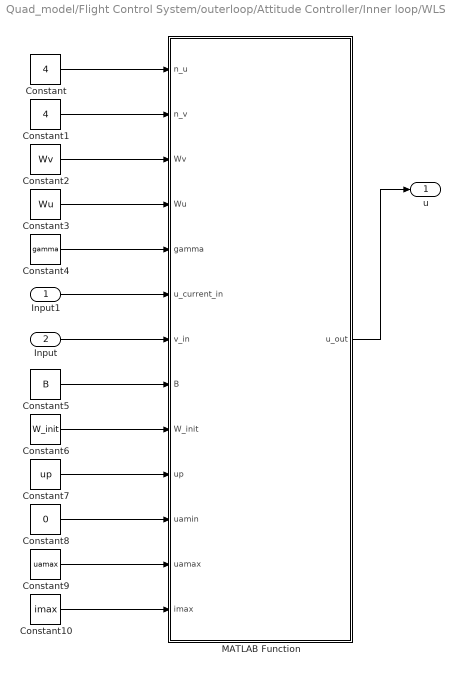
== system Quad_model/Flight Control System/outerloop/Attitude Controller/Inner loop/WLS ==
  Input1 : Inport
  Input : Inport  Port=2
  Constant : Constant  Value=4
  Constant1 : Constant  Value=4
  Constant10 : Constant  Value=imax
  Constant2 : Constant  Value=Wv
  Constant3 : Constant  Value=Wu
  Constant4 : Constant  Value=gamma
  Constant5 : Constant  Value=B
  Constant6 : Constant  Value=W_init
  Constant7 : Constant  Value=up
  Constant8 : Constant  Value=0
  Constant9 : Constant  Value=uamax
  MATLAB Function : MATLAB Function  TreatAsAtomicUnit=on
  u : Outport
  wires:
  Constant8/1 -> MATLAB Function/11(uamin)
  Constant4/1 -> MATLAB Function/5(gamma)
  Constant/1 -> MATLAB Function/1(n_u)
  MATLAB Function/1(u_out) -> u/1
  Constant5/1 -> MATLAB Function/8(B)
  Constant9/1 -> MATLAB Function/12(uamax)
  Constant6/1 -> MATLAB Function/9(W_init)
  Constant10/1 -> MATLAB Function/13(imax)
  Constant1/1 -> MATLAB Function/2(n_v)
  Constant2/1 -> MATLAB Function/3(Wv)
  Constant3/1 -> MATLAB Function/4(Wu)
  Constant7/1 -> MATLAB Function/10(up)
  Input1/1 -> MATLAB Function/6(u_current_in)
  Input/1 -> MATLAB Function/7(v_in)

== matlab function Quad_model/Flight Control System/outerloop/Simulation Environment/Drag Approximation/MATLAB Function1 ==
  data: N input; y output; E input
function y = traj_ang(N,E)
a = atan2(E,N);
y = a;
end

== matlab function Quad_model/Flight Control System/outerloop/WLS/MATLAB Function ==
  data: n_u input size=1; u_out output size=[3 1]; n_v input size=1; Wv input size=3; Wu input size=3; gamma input size=1; u_current_in input size=[3 1]; v_in input size=3; B input; W_init input size=[1 3]; up input size=3; uamin input size=[1 3]; uamax input size=[1 3]; imax input size=1
function u_out  = wls(n_u,n_v,Wv,Wu,gamma,u_current_in,v_in,B,W_init,up,uamin,uamax,imax)
%UNTITLED2 Summary of this function goes here
%   Detailed explanation goes here
%u_current = u_current.';
v = v_in.';
disp('v_in')
disp(v_in)
%coder.varsize('u_current');
u_current = u_current_in.';
disp(size(u_current))
disp(size(uamin))
disp(size(min((uamin-u_current),0)))
umin = min((uamin-u_current),0);%[52,52,52,52];
umax = max((uamax-u_current),0);%[733,733,733,733];
u_guess = 0.5 * (umax-umin);
up = [-u_current(1), -u_current(2), umin(3)];
break_flag = false;
n_u = 3; % size control input
n_v = 3; % size control objective
n_c = n_u+n_v;

A = zeros(n_c,n_u);
A_free = zeros(n_c,n_u);

b = zeros(1,n_c);
d = zeros(1,n_c);

free_index = zeros(1,n_u);
free_index_lookup = zeros(1,n_u);
n_free = 0; %0
free_chk = -1;
iter = 0;
p_free = zeros(1,n_u);
p = zeros(1,n_u);

infeasible_index = zeros(1,n_u);
n_infeasible = 0;
lambda = zeros(1,n_u);
W = zeros(1,n_u);
u_opt = zeros(1,n_u);

u = u_guess;
W = W_init;
free_index_lookup = ones(1,n_u) * -1;

for i=1:n_u
    if W(1,i)== 0
        n_free = n_free+1;
        free_index_lookup(i) = n_free;
        free_index(n_free)= i;
        
    end
end

for i = 1:n_v
    b(i) = gamma * Wv(i) * v(i);
    d(i) = b(i);
    for j =1:n_u
        A(i,j) = gamma * Wv(i) * B(i,j);
        d(i) = d(i) - A(i,j) * u(j);
    end  
end

for i = (n_v+1):n_c
    A(i,:) = zeros(1,n_u);
    A(i,i-n_v) = Wu(i-n_v);
    b(i) = Wu(i-n_v)*up(i-n_v);
    d(i) = b(i) - A(i,i-n_v)* u(i-n_v);

end
while (iter < imax)
    %fprintf('iter = %i \n',iter)
    disp(iter)
    p = zeros(1,n_u);
    u_opt = u;
    u_check = zeros(1,n_u);

    if free_chk ~= n_free
        for i =1:n_c
            for j=1:n_free
                A_free(i,j) = A(i,free_index(j));
            end
        end
        free_chk = n_free;
    end

    if n_free>0
        p_free= (A_free\d.').';
    else
        disp('no free actuator')
        break
    end

    for i =1:n_free
        p(free_index(i)) = p_free(i);
        u_opt(free_index(i)) = u_opt(free_index(i)) + p_free(i);
    end

    n_infeasible = 0;
    for i = 1:n_u
        if u_opt(i)>= (umax(i)+1) || u_opt(i)<= (umin(i)-1)
            %disp('INFEASIBLE')
            n_infeasible = n_infeasible+1;
            infeasible_index(n_infeasible) = i;
            if u_opt(i)<= (umin(i))
                u_check(i)= 1;
            end
            
        end
    end
    
    if n_infeasible == 0
        u = u_opt;%[1,1,1,1];% HELOOOOOO
        lambda = zeros(1,n_u);
        for i =1:n_c
            for k =1:n_free
                d(i) = d(i) - A_free(i,k)*p_free(k);
            end
            for k =1:n_u
                lambda(k) = lambda(k)+A(i,k)*d(i);
            end
        end
        break_flag = true;
        %disp(lambda)
        for i = 1:n_u
            lambda(i) = lambda(i)*W(1,i);
            %disp('check')
            %disp(lambda(i))
            if lambda(i) < 0
                %disp('check 2')
                break_flag = false;
                W(1,i) = 0;

                if free_index_lookup(i) <0
                    n_free =n_free +1;
                    free_index_lookup(i) = n_free;
                    free_index(n_free) = i;
                    
                end
            end
        end

        if break_flag
            output = iter;
            break
        end
    else
        

        alpha = inf;
        alpha_tmp = 0;
        id_alpha = 1;

        for i = 1:n_free
            id=free_index(i);
            %disp('p(id)')
            %disp(p(id))
            if abs(p(id))>1.1920928955078125e-7%0
                %disp('alpha_check_true')
                %disp(id)
                %alpha_tmp = (p(id)<0)*(umin(id)-u(id))/p(id)+ (1-(p(id)<0))*(umax(id)-u(id))/p(id);
                alpha_tmp = (u_check(id))*(umin(id)-u(id))/p(id)+ (1-u_check(id))*(umax(id)-u(id))/p(id);
                %disp(alpha_tmp)
            else
                %disp('alpha_check_false')
                %disp(id)
                alpha_tmp = inf;
            end
            if alpha_tmp < alpha %ABSSSSSSS
                %disp('alpha')
                %disp(id)
                alpha =alpha_tmp;
                id_alpha = id;
            end
        end
        
        for i =1:n_u
            u(i)=u(i)+alpha*p(i);
        end


        for i =1:n_c
            for k =1:n_free
                d(i) = d(i) - A_free(i,k)*alpha*p_free(k);
            end
        end
        %disp('free index lookup')
        %disp(free_index_lookup)
        %disp(free_index)
        %disp(id_alpha)

        %W(1,id_alpha) = (p(id_alpha)>0) *1 + (1- (p(id_alpha)>0)) * -1;
        W(id_alpha) = (u_check(id_alpha)<=0) *1 + (1-(u_check(id_alpha)<=0)) * -1;
        %disp('nfree')
        %disp(n_free)
        free_index(free_index_lookup(id_alpha)) = free_index(n_free);
        n_free = n_free -1;
        free_index_lookup(free_index(free_index_lookup(id_alpha))) = free_index_lookup(id_alpha);
        free_index_lookup(id_alpha) = -1 ;
        
    end 
    output = -1;
    
    iter = iter +1;
end
% if output == -1
%     disp('all saturated')
% else
%     disp('Great Sucscess')
%     disp(u_current+u)
% end
disp('u')
disp(u)
disp('u_tot')
disp(u_current+u)
u_out = u.';

%u = u.';
end

== matlab function Quad_model/Flight Control System/outerloop/Gn_calculator/Gn_inv ==
  data: T input; phi input; theta input; psi input; Gn_inv data_store_memory
function Gn_inv(T,phi,theta, psi)
%#codegen

%    This function was generated by the Symbolic Math Toolbox version 9.0.
%    02-Jan-2022 12:29:17
global Gn_inv;
t2 = cos(phi);
t3 = cos(psi);
t4 = cos(theta);
t5 = sin(phi);
t6 = sin(psi);
t7 = sin(theta);
t8 = 1.0./T;
t9 = 1.0./t2;
Gn_inv = reshape([t8.*(t2.*t6-t3.*t5.*t7),t3.*t4.*t8.*t9,t5.*t6+t2.*t3.*t7,-t8.*(t2.*t3+t5.*t6.*t7),t4.*t6.*t8.*t9,-t3.*t5+t2.*t6.*t7,-t4.*t5.*t8,-t7.*t8.*t9,t2.*t4],[3,3]);

== matlab function Quad_model/Flight Control System/outerloop/Gn_calculator/Gn ==
  data: T input; phi input; theta input; psi input; Gn data_store_memory
function Gn(T,phi,theta,psi)
%#codegen

%    This function was generated by the Symbolic Math Toolbox version 9.0.
%    02-Jan-2022 12:18:38
global Gn;
t2 = cos(phi);
t3 = cos(psi);
t4 = cos(theta);
t5 = sin(phi);
t6 = sin(psi);
t7 = sin(theta);
Gn = reshape([T.*(t2.*t6-t3.*t5.*t7),-T.*(t2.*t3+t5.*t6.*t7),-T.*t4.*t5,T.*t2.*t3.*t4,T.*t2.*t4.*t6,-T.*t2.*t7,t5.*t6+t2.*t3.*t7,-t3.*t5+t2.*t6.*t7,t2.*t4],[3,3]);

== matlab function Quad_model/Flight Control System/outerloop/Attitude Controller/Inner loop/WLS/MATLAB Function ==
  data: n_u input size=1; u_out output size=[4 1]; n_v input size=1; Wv input size=4; Wu input size=4; gamma input size=1; u_current_in input size=[4 1]; v_in input size=4; B input; W_init input size=[1 4]; up input size=4; uamin input size=1; uamax input size=1; imax input size=1
function u_out  = wls(n_u,n_v,Wv,Wu,gamma,u_current_in,v_in,B,W_init,up,uamin,uamax,imax)
%UNTITLED2 Summary of this function goes here
%   Detailed explanation goes here
%u_current = u_current.';
v = v_in.';
disp('v_in')
disp(v_in)
%coder.varsize('u_current');
u_current = u_current_in.';
umin = min((uamin-u_current),0);%[52,52,52,52];
umax = max((uamax-u_current),0);%[733,733,733,733];
u_guess = 0.5 * (umax-umin);
up = umin;
break_flag = false;
n_u = 4; % size control input
n_v = 4; % size control objective
n_c = n_u+n_v;

A = zeros(n_c,n_u);
A_free = zeros(n_c,n_u);

b = zeros(1,n_c);
d = zeros(1,n_c);

free_index = zeros(1,n_u);
free_index_lookup = zeros(1,n_u);
n_free = 0; %0
free_chk = -1;
iter = 0;
p_free = zeros(1,n_u);
p = zeros(1,n_u);

infeasible_index = zeros(1,n_u);
n_infeasible = 0;
lambda = zeros(1,n_u);
W = zeros(1,n_u);
u_opt = zeros(1,n_u);

u = u_guess;
W = W_init;
free_index_lookup = ones(1,n_u) * -1;

for i=1:n_u
    if W(1,i)== 0
        n_free = n_free+1;
        free_index_lookup(i) = n_free;
        free_index(n_free)= i;
        
    end
end

for i = 1:n_v
    b(i) = gamma * Wv(i) * v(i);
    d(i) = b(i);
    for j =1:n_u
        A(i,j) = gamma * Wv(i) * B(i,j);
        d(i) = d(i) - A(i,j) * u(j);
    end  
end

for i = (n_v+1):n_c
    A(i,:) = zeros(1,n_u);
    A(i,i-n_v) = Wu(i-n_v);
    b(i) = Wu(i-n_v)*up(i-n_v);
    d(i) = b(i) - A(i,i-n_v)* u(i-n_v);

end
while (iter < imax)
    %fprintf('iter = %i \n',iter)
    disp(iter)
    p = zeros(1,n_u);
    u_opt = u;
    u_check = zeros(1,n_u);

    if free_chk ~= n_free
        for i =1:n_c
            for j=1:n_free
                A_free(i,j) = A(i,free_index(j));
            end
        end
        free_chk = n_free;
    end

    if n_free>0
        p_free= (A_free\d.').';
    else
        disp('no free actuator')
        break
    end

    for i =1:n_free
        p(free_index(i)) = p_free(i);
        u_opt(free_index(i)) = u_opt(free_index(i)) + p_free(i);
    end

    n_infeasible = 0;
    for i = 1:n_u
        if u_opt(i)>= (umax(i)+1) || u_opt(i)<= (umin(i)-1)
            %disp('INFEASIBLE')
            n_infeasible = n_infeasible+1;
            infeasible_index(n_infeasible) = i;
            if u_opt(i)<= (umin(i))
                u_check(i)= 1;
            end
            
        end
    end
    
    if n_infeasible == 0
        u = u_opt;%[1,1,1,1];% HELOOOOOO
        lambda = zeros(1,n_u);
        for i =1:n_c
            for k =1:n_free
                d(i) = d(i) - A_free(i,k)*p_free(k);
            end
            for k =1:n_u
                lambda(k) = lambda(k)+A(i,k)*d(i);
            end
        end
        break_flag = true;
        %disp(lambda)
        for i = 1:n_u
            lambda(i) = lambda(i)*W(1,i);
            %disp('check')
            %disp(lambda(i))
            if lambda(i) < 0
                %disp('check 2')
                break_flag = false;
                W(1,i) = 0;

                if free_index_lookup(i) <0
                    n_free =n_free +1;
                    free_index_lookup(i) = n_free;
                    free_index(n_free) = i;
                    
                end
            end
        end

        if break_flag
            output = iter;
            break
        end
    else
        

        alpha = inf;
        alpha_tmp = 0;
        id_alpha = 1;

        for i = 1:n_free
            id=free_index(i);
            %disp('p(id)')
            %disp(p(id))
            if abs(p(id))>1.1920928955078125e-7%0
                %disp('alpha_check_true')
                %disp(id)
                %alpha_tmp = (p(id)<0)*(umin(id)-u(id))/p(id)+ (1-(p(id)<0))*(umax(id)-u(id))/p(id);
                alpha_tmp = (u_check(id))*(umin(id)-u(id))/p(id)+ (1-u_check(id))*(umax(id)-u(id))/p(id);
                %disp(alpha_tmp)
            else
                %disp('alpha_check_false')
                %disp(id)
                alpha_tmp = inf;
            end
            if alpha_tmp < alpha %ABSSSSSSS
                %disp('alpha')
                %disp(id)
                alpha =alpha_tmp;
                id_alpha = id;
            end
        end
        
        for i =1:n_u
            u(i)=u(i)+alpha*p(i);
        end


        for i =1:n_c
            for k =1:n_free
                d(i) = d(i) - A_free(i,k)*alpha*p_free(k);
            end
        end
        %disp('free index lookup')
        %disp(free_index_lookup)
        %disp(free_index)
        %disp(id_alpha)

        %W(1,id_alpha) = (p(id_alpha)>0) *1 + (1- (p(id_alpha)>0)) * -1;
        W(id_alpha) = (u_check(id_alpha)<=0) *1 + (1-(u_check(id_alpha)<=0)) * -1;
        %disp('nfree')
        %disp(n_free)
        free_index(free_index_lookup(id_alpha)) = free_index(n_free);
        n_free = n_free -1;
        free_index_lookup(free_index(free_index_lookup(id_alpha))) = free_index_lookup(id_alpha);
        free_index_lookup(id_alpha) = -1 ;
        
    end 
    output = -1;
    
    iter = iter +1;
end
% if output == -1
%     disp('all saturated')
% else
%     disp('Great Sucscess')
%     disp(u_current+u)
% end
disp('u')
disp(u)
disp('u_tot')
disp(u_current+u)
u_out = u.';

%u = u.';
end

== matlab function Quad_model/Flight Control System/outerloop/Heading controller/MATLAB Function ==
  data: u input; omega output; phi input; lim input
function omega = fcn(u,phi,lim)
%Sideslip controller
if u > lim
    omega = 9.81/u*tan(phi);
else
    omega = 0;
end

== matlab function Quad_model/Flight Control System/outerloop/Heading controller/MATLAB Function1 ==
  data: N input; y output; E input; u input; lim input
function y = traj_ang(N,E,u,lim)
a = atan2(E,N);
if u > lim
    y = a;
else
    y = 0;
end

== matlab function Quad_model/Flight Control System/outerloop/Simulation Environment/Drag Approximation/MATLAB Function ==
  data: cd input; rho input; u input; F_drag output; A input; trj input
function F_drag = fcn(cd,rho,u,A,trj)
drag = 0.5*rho*u^2*A*cd;
F_drag = [-cos(trj); -sin(trj)]*drag;

== matlab function Quad_model/Flight Control System/outerloop/Simulation Environment/Tn ==
  data: phi input; theta input; Tn output; psi input; T input
function Tn = Tn(phi,theta,psi,T)
%#codegen

%    This function was generated by the Symbolic Math Toolbox version 9.0.
%    28-Jan-2022 12:03:54

t2 = cos(phi);
t3 = cos(psi);
t4 = sin(phi);
t5 = sin(psi);
t6 = sin(theta);
Tn = [T.*(t4.*t5+t2.*t3.*t6);-T.*(t3.*t4-t2.*t5.*t6);T.*t2.*cos(theta)];
